simulink library "CAV1553_PCI_BC"  (Simulink 7.8)
settings: Solver=ode5  SolverMode=SingleTasking  StartTime=0.0  StopTime=Inf  FixedStep=0.001  RelTol=1e-3
settings Model: Creator=Administrator  LastModifiedBy=Administrator

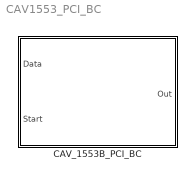
== system CAV1553_PCI_BC ==
  CAV_1553B_PCI_BC : Subsystem  mask(CAV_1553_BC){pci_id=0, chan_id=0, bc_identifer=0, bc_num=1, bus_ctrl_op=BCRT, bus_num=Bus A, sourcert_add=0, sourcert_subadd=0, destrt_add=0, destrt_subadd=0, last_bc=0, is_first_bc=0}
      mask prompts: pci_id "PCI ID"; chan_id "Channel ID"; bc_identifer "BC Identifier"; bc_num "BC Number"; bus_ctrl_op "Bus control operation"; bus_num "Bus Number"; sourcert_add "Source Remote Terminal"; sourcert_subadd "Source Sub-Address"; destrt_add "Destination Remote Terminal"; destrt_subadd "Destination Sub-Address"; last_bc "Data Count(0 for 32 word)"; is_first_bc "Data Count"
      mask help:
      | This block is used for BC .It can control all of the act about BC .
      | If you have ONLY ONE BC block ,the BC Identifier you can set anyone.
      | But if you have MORE THAN ONE BC block ,the BC Identifier should be set continuously ,for example you have THREE bc block ,the BC Identifier
      | should be from 0 to 2 .For details ,reference with the docs .
      mask init:
      | if( bus_ctrl_op == 1)
      |     if(bus_num == 1)
      | 		displayblock=sprintf('\n CAV 1553B BC \nBC:%d\nBC-RT\nBus A\nPCI Id: %d\nChannel Id: %d\n RT: %d-%d\n ',bc_identifer, pci_id, chan_id,destrt_add,destrt_subadd);
      |     elseif(bus_num == 2)
      | 		displayblock=sprintf('\n CAV 1553B BC \nBC:%d\nBC-RT\nBus B\nPCI Id: %d\nChannel Id: %d\nDestination RT: %d\nDestination Sub-Address :%d\n ',bc_identifer, pci_id, chan_id,destrt_add,destrt_subadd);
      |     else
      | 		displayblock=sprintf('\n CAV 1553B BC \nBC:%d\nBC-RT\nBus Error\nPCI Id: %d\nChannel Id: %d\nDestination RT: %d\nDestination Sub-Address :%d\n ',bc_identifer, pci_id, chan_id,destrt_add,destrt_subadd);
      |     end
      | elseif (bus_ctrl_op == 2)
      |     if(bus_num == 1)
      |         displayblock=sprintf('\n CAV 1553B BC \nBC:%d\nRT-RT\nBus A\nPCI Id: %d\nChannel Id: %d\nRT Add: %d-%d\nSub RT: %d-%d\n',bc_identifer, pci_id, chan_id,sourcert_add,sourcert_subadd,destrt_add,destrt_subadd);
      |     elseif(bus_num == 2)
      |         displayblock=sprintf('\n CAV 1553B BC \nBC:%d\nRT-RT\nBus B\nPCI Id: %d\nChannel Id: %d\nRT Add: %d-%d\nSub RT: %d-%d\n',bc_identifer, pci_id, chan_id,sourcert_add,sourcert_subadd,destrt_add,destrt_subadd);
      |     else
      |         displayblock=sprintf('\n CAV 1553B BC \nBC:%d\nRT-RT\nBus ERROR\nPCI Id: %d\nChannel Id: %d\nRT Add: %d-%d\nSub RT: %d-%d\n',bc_identifer, pci_id, chan_id,sourcert_add,sourcert_subadd,destrt_add,destrt_subadd);
      |     end
      | elseif (bus_ctrl_op == 3)
      |     if(bus_num == 1)
      |         displayblock=sprintf('\n CAV 1553B BC \nBC:%d\nBCRT_BROADCAST\nBus A\nPCI Id: %d\nChannel Id: %d\nDestination Sub-Address: %d\n', bc_identifer,pci_id, chan_id,destrt_subadd);
      |     elseif(bus_num == 2)
      |         displayblock=sprintf('\n CAV 1553B BC \nBC:%d\nBCRT_BROADCAST\nBus B\nPCI Id: %d\nChannel Id: %d\nDestination Sub-Address: %d\n',bc_identifer, pci_id, chan_id,destrt_subadd);
      |     else
      |         displayblock=sprintf('\n CAV 1553B BC \nBC:%d\nBCRT_BROADCAST\nBus Error\nPCI Id: %d\nChannel Id: %d\nDestination Sub-Address: %d\n',bc_identifer, pci_id, chan_id,destrt_subadd);
      |     end
      | elseif (bus_ctrl_op == 4)
      |     if(bus_num == 1)
      |         displayblock=sprintf('\n CAV 1553B BC \nBC:%d\nRTRT_BROADCAST\nBus A\nPCI Id: %d\nChannel Id: %d\nRT Add: %d-%d\n Destination Sub-Address:%d\n',bc_identifer, pci_id, chan_id,sourcert_add,sourcert_subadd,destrt_subadd);
      |     elseif(bus_num == 2)
      |         displayblock=sprintf('\n CAV 1553B BC \nBC:%d\nRTRT_BROADCAST\nBus B\nPCI Id: %d\nChannel Id: %d\nRT Add: %d-%d\n Destination Sub-Address:%d\n',bc_identifer, pci_id, chan_id,sourcert_add,sourcert_subadd,destrt_subadd);
      |     else
      |         displayblock=sprintf('\n CAV 1553B BC \nBC:%d\nRTRT_BROADCAST\nBus Error\nPCI Id: %d\nChannel Id: %d\nRT Add: %d-%d\n Destination Sub-Address:%d\n', bc_identifer,pci_id, chan_id,sourcert_add,sourcert_subadd,destrt_subadd);
      |     end
      | else
      |     if(bus_num == 1)
      |         displayblock=sprintf('\n CAV 1553B BC \nBC:%d\nRTBC\nBus A\nPCI Id: %d\nChannel Id: %d\nSourceRT Add: %d-%d\n ', bc_identifer,pci_id, chan_id,sourcert_add,sourcert_subadd);
      |     elseif(bus_num == 2)
      |         displayblock=sprintf('\n CAV 1553B BC \nBC:%d\nRTBC\nBus B\nPCI Id: %d\nChannel Id: %d\nSourceRT Add: %d-%d\n ', bc_identifer,pci_id, chan_id,sourcert_add,sourcert_subadd);
      |     else
      |         displayblock=sprintf('\n CAV 1553B BC \nBC:%d\nRTBC\nBus Err\nPCI Id: %d\nChannel Id: %d\nSourceRT Add: %d-%d\n ',bc_identifer, pci_id, chan_id,sourcert_add,sourcert_subadd);
      |     end
      | end
      mask StyleString: edit,edit,edit,edit,popup(BCRT|RTRT|BCRT_BROADCAST|RTRT_BROADCAST|RTBC),popup(Bus A|Bus B),edit,edit,edit,edit,edit,edit
      mask CallbackString:
      | ||
      | ||bco = get_param(gcb,'bus_ctrl_op');
      | 
      | if(strcmp(bco,'BCRT')),
      |     set_param(gcb,'MaskEnables',{'on';'on';'on';'on';'on';'on';'off';'off';'on';'on';'on';'off'}),
      | elseif(strcmp(bco,'RTRT')),
      |     set_param(gcb,'MaskEnables',{'on';'on';'on';'on';'on';'on';'on';'on';'on';'on';'on';'off'}),
      | elseif(strcmp(bco,'BCRT_BROADCAST')),
      |     set_param(gcb,'MaskEnables',{'on';'on';'on';'on';'on';'on';'off';'on';'on';'on';'on';'off'}),
      | elseif(strcmp(bco,'RTRT_BROADCAST')),
      |     set_param(gcb,'MaskEnables',{'on';'on';'on';'on';'on';'on';'on';'on';'off';'on';'on';'off'}),
      | else
      |     set_param(gcb,'MaskEnables',{'on';'on';'on';'on';'on';'on';'on';'on';'off';'off';'on';'off'}),
      | end
      |  |||||||
      mask Display: disp(displayblock);

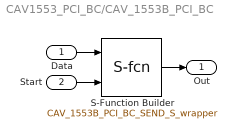
== system CAV1553_PCI_BC/CAV_1553B_PCI_BC ==
  Data : Inport
  Start : Inport  Port=2
  S-Function Builder : S-Function  InitFcn=try, set_param(gcb,'FunctionName','CAV_1553B_PCI_BC_SEND_S_wrapper'), end  FunctionName=CAV_1553B_PCI_BC_SEND_S_wrapper  Parameters=pci_id,chan_id,is_first_bc,bc_num,bc_identifer,bus_ctrl_op,bus_num,sourcert_add,sourcert_subadd,destrt_add,destrt_subadd,last_bc  WizardData=DataTag0  EnableBusSupport=off  mask(S-Function Builder){}
      mask help: Simulink:masks:SFunctionBuilder_MD
      mask init:
      | val = [[.9  0.75 0.75 1 1 .9 .9 1]',[1 1 0.75 0.75 .9 .9 1 .9]'];try , sys = get_param(gcb,'SfunBuilderFcnName');if isempty(sys), sys = get_param(gcb,'FunctionName'); end,catch, sys = get_param(gcb,'FunctionName'); end
      settings: CopyFcn=set_param(gcbh,'LinkStatus','none')  PreSaveFcn=try, set_param(gcb,'FunctionName','CAV_1553B_PCI_BC_SEND_S_wrapper'), end  OpenFcn=sfunctionwizard(gcbh)
      mask Display: plot(val(:,1),val(:,2)),disp(sys), port_label('input',1,'u0'), port_label('input',2,'u1'), port_label('output',1,'y0')
  Out : Outport
  wires:
  Start/1 -> S-Function Builder/2
  S-Function Builder/1 -> Out/1
  Data/1 -> S-Function Builder/1
